simulink model "PIcontrol_smo"  (R2022a)
settings: Solver=VariableStepAuto  StartTime=0.0  StopTime=2.5  MaxStep=1e-4  MinStep=1e-6  RelTol=1e-6
undefined symbols (not defined in the file or in its folder): DiscIntNeverNeededParam
libraries: spsIGBTDiodeLib x6, simulink x3, mcbcontrolslib x1, spsDCVoltageSourceLib x1, spsPermanentMagnetSynchronousMachineLib x1, spspowerguiLib x1
settings Model: Creator=18527  LastModifiedBy=18527
settings SolverCC: ZeroCrossAlgorithm=Adaptive
settings DebuggingCC: IgnoredZcDiagnostic=none

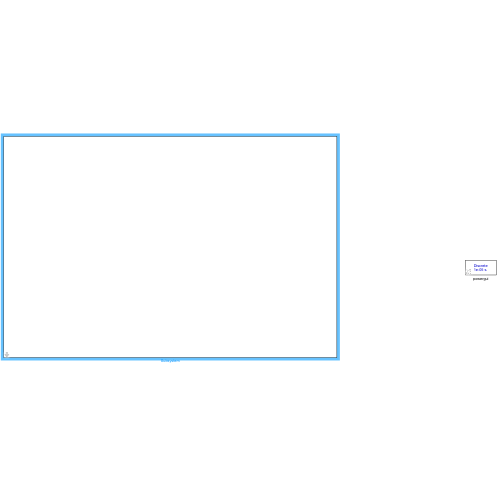
[thumbnail: Simulink's stored preview of the top-level diagram]
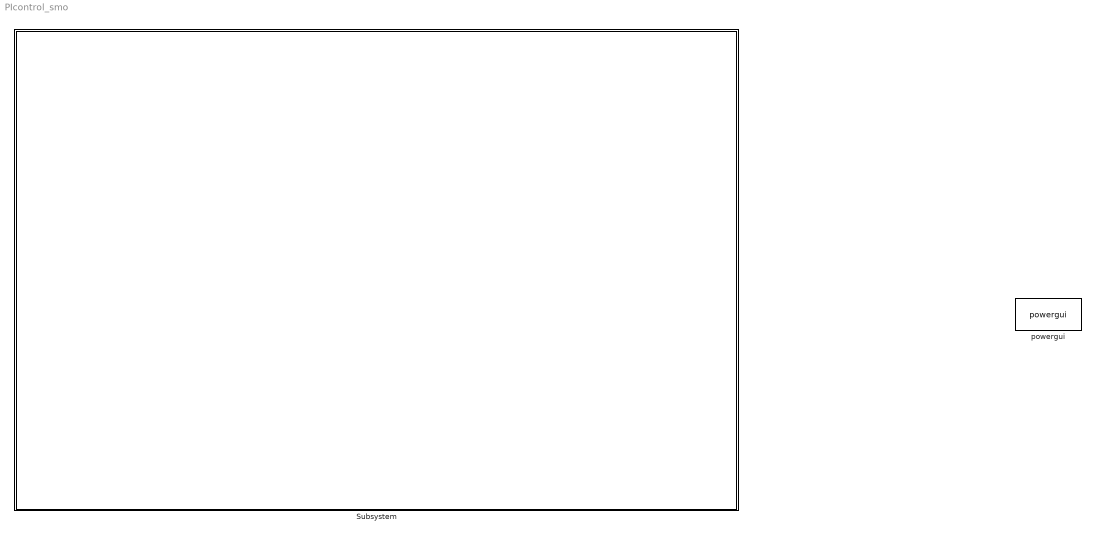
== system PIcontrol_smo ==
  Subsystem : Subsystem  mask{Pn=4, Ld=5.25e-3, Lq=12e-3, R=0.958, J=0.003, B=0.008, Phi=0.1827, OPL_Time=2, Switch_Speed=800}
      mask prompts: Pn "极对数"; Ld "定子电感"; Lq "定子电感"; R "定子电阻"; J "转动惯量"; B "阻尼系数"; Phi "磁链"; OPL_Time "开环时间"; Switch_Speed "切闭环速度"
      mask DialogControl ParameterGroupVar Prompt: 参数
  powergui : spspowerguiLib/powergui  Priority=1  SimulationMode=Discrete  SampleTime=1e-5  frequency=60  Iterations=50  frequencyindice=0  Pbase=100e6  ErrMax=1e-4  UnitsV=kV  UnitsW=MW  buscounter=0  FunctionMessages=off  echomessages=off  EnableUseOfTLC=off  CurrentSourceSwitches=off  DisableSnubberDevices=off  DisableRonSwitches=off  DisableVfSwitches=off  DisplayEquations=off  AutomaticDiscreteSolvers=off  SolverType=Tustin/Backward Euler (TBE)  Interpol=off  ExternalGateDelay=off  methode=off  Ts=100  x0status=blocks  SPID=on  SwTol=0  HookPort=off  NonlinearTolerance=1e-4  nMaxIteration=100  ContinueOnMaxIteration=off  RestoreLinks=warning  ResistiveCurrentMeasurement=off  Frange=[0:2:500]  Ylog=off  Xlog=on  ShowGrid=off  save=off  variable=ZData  structure=0  ZoomFFT=off  StartTime=0.0  cycles=1  DisplayStyle=1  fundamental=60  FreqAxis=off  MaxFrequency=1000  frequencyindicesteady=1  RmsSteady=1  display=off

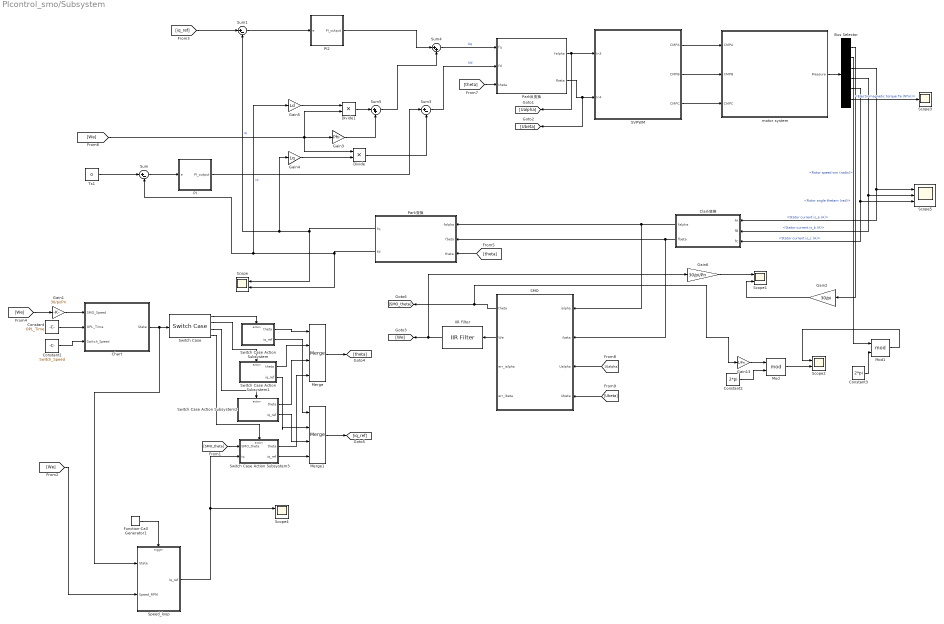
== system PIcontrol_smo/Subsystem ==
  Bus Selector : BusSelector  OutputSignals=Rotor speed wm (rad/s),Rotor angle thetam (rad),Stator current is_a (A),Stator current is_b (A),Stator current is_c (A),Electromagnetic torque Te (N*m)
  Chart : Stateflow chart  TreatAsAtomicUnit=on
  Clark变换 : Subsystem
  Constant : Constant  Value=OPL_Time
  Constant1 : Constant  Value=Switch_Speed
  Constant2 : Constant  Value=2*pi
  Constant3 : Constant  Value=2*pi
  Divide : Product  Inputs=**
  Divide1 : Product  Inputs=**
  Function-Call Generator1 : simulink/Ports & Subsystems/Function-Call Generator  sample_time=0.002  numberOfIterations=1  DisallowWideOutput=off
  Gain1 : Gain  Gain=30/pi/Pn
  Gain13 : Gain  Gain=1/Pn
  Gain2 : Gain  Gain=30/pi
  Gain3 : Gain  Gain=Phi
  Gain4 : Gain  Gain=Lq
  Gain5 : Gain  Gain=Ld
  Gain6 : Gain  Gain=30/pi/Pn
  IIR Filter : mcbcontrolslib/IIR Filter  VariantControl=Low Pass Filter  VariantSelect=Low-pass  Filter_constant=0.0008  advancedSettings=off  Ts=6e-6  cutOff_freq=21.2376
      settings: SourceProductBaseCode=MT
  Merge : Merge  Inputs=4
  Merge1 : Merge  Inputs=4
  Mod : Math  Operator=mod
  Mod1 : Math  Operator=mod
  PI : Subsystem  mask{Kp=Ld*4000/2, Ki=R*4000/2}
      mask prompts: Kp "比例"; Ki "积分"
      mask DialogControl ParameterGroupVar Prompt: 参数
  PI2 : Subsystem  mask{Kp=Lq*4000/2, Ki=R*4000/2}
      mask prompts: Kp "比例"; Ki "积分"
      mask DialogControl ParameterGroupVar Prompt: 参数
  Park反变换 : Subsystem
  Park变换 : Subsystem
  SMO : Subsystem
  SVPWM : Subsystem
  Scope{,1..2,4} (4 alike) : Scope  NumInputPorts=2
  Scope3 : Scope
  Scope5 : Scope  NumInputPorts=3
  Speed_loop : Subsystem
      settings: RTWSystemCode=Nonreusable function  RTWFcnNameOpts=Use subsystem name
  Sum : Sum  Inputs=|+-
  Sum1 : Sum  Inputs=|+-
  Sum3 : Sum  Inputs=|+-
  Sum4 : Sum  Inputs=|++
  Sum5 : Sum  Inputs=|++
  Switch Case : SwitchCase  CaseConditions={1,2,3,4}  ShowDefaultCase=off
  Switch Case Action Subsystem : Subsystem  TreatAsAtomicUnit=on
  Switch Case Action Subsystem1 : Subsystem  TreatAsAtomicUnit=on
  Switch Case Action Subsystem2 : Subsystem  TreatAsAtomicUnit=on
  Switch Case Action Subsystem3 : Subsystem  TreatAsAtomicUnit=on
  Ts1 : Constant  Value=0
  motor system : Subsystem
  wires:
  Sum1/1 -> PI2/1(e)
  Sum4/1 -> Park反变换/1(fq)  "Uq"
  motor system/1(Measure) -> Bus Selector/1
  PI2/1(PI_output) -> Sum4/1
  Park反变换/1(falpha) -> SVPWM/1(In3), [Ualpha]
  Park反变换/2(fbeta) -> [Ubeta], SVPWM/2(In4)
  SVPWM/1(CMPA) -> motor system/1(CMPA)
  SVPWM/2(CMPB) -> motor system/2(CMPB)
  SVPWM/3(CMPC) -> motor system/3(CMPC)
  Bus Selector/3 -> Scope5/1, Clark变换/1(fA)  "<Stator current is_a (A)>"
  Bus Selector/4 -> Clark变换/2(fB), Scope5/2  "<Stator current is_b (A)>"
  Bus Selector/5 -> Scope5/3, Clark变换/3(fC)  "<Stator current is_c (A)>"
  Clark变换/1(falpha) -> SMO/1(ialpha), Park变换/1(falpha)
  Clark变换/2(fbeta) -> SMO/2(ibeta), Park变换/2(fbeta)
  [Ubeta] -> SMO/4(Ubeta)
  [Ualpha] -> SMO/3(Ualpha)
  Gain5/1 -> Divide1/1
  [We] -> Divide1/2, Gain3/1, Divide/1
  PI/1(PI_output) -> Sum3/1
  Ts1/1 -> Sum/1
  Sum/1 -> PI/1(e)
  SMO/2(We) -> IIR Filter/1
  Gain4/1 -> Divide/2
  Park变换/2(fd) -> Scope/2, Gain5/1, Sum/2  "id"
  Park变换/1(fq) -> Scope/1, Gain4/1, Sum1/2  "iq"
  Divide1/1 -> Sum5/1
  Gain3/1 -> Sum5/2
  Divide/1 -> Sum3/2
  Sum5/1 -> Sum4/2
  Sum3/1 -> Park反变换/2(fd)  "Ud"
  Bus Selector/1 -> Gain2/1  "<Rotor speed wm (rad/s)>"
  Gain2/1 -> Scope1/2
  Gain6/1 -> Scope1/1
  SMO/1(theta) -> Gain13/1, [SMO_theta]
  Bus Selector/2 -> Mod1/1  "<Rotor angle thetam (rad)>"
  Bus Selector/6 -> Scope3/1  "<Electromagnetic torque Te (N*m)>"
  Switch Case/1 -> Switch Case Action Subsystem/Action
  Switch Case Action Subsystem/1(theta) -> Merge/1
  Switch Case/2 -> Switch Case Action Subsystem1/Action
  Switch Case/3 -> Switch Case Action Subsystem2/Action
  Switch Case Action Subsystem1/1(theta) -> Merge/2
  Switch Case Action Subsystem2/1(theta) -> Merge/3
  Switch Case Action Subsystem3/1(theta) -> Merge/4
  Switch Case Action Subsystem/2(iq_ref) -> Merge1/1
  Switch Case Action Subsystem1/2(iq_ref) -> Merge1/2
  Switch Case Action Subsystem2/2(iq_ref) -> Merge1/3
  Switch Case Action Subsystem3/2(iq_ref) -> Merge1/4
  Merge/1 -> [theta]
  Merge1/1 -> [iq_ref]
  IIR Filter/1 -> Gain6/1, [We]
  [SMO_theta] -> Switch Case Action Subsystem3/1(SMO_theta)
  [iq_ref] -> Sum1/1
  Switch Case/4 -> Switch Case Action Subsystem3/Action
  [We] -> Speed_loop/2(Speed_RPM)
  Chart/1(State) -> Speed_loop/1(State), Switch Case/1
  [We] -> Gain1/1
  Gain1/1 -> Chart/1(SMO_Speed)
  Constant/1 -> Chart/2(OPL_Time)
  Constant1/1 -> Chart/3(Switch_Speed)
  [theta] -> Park变换/3(theta)
  [theta] -> Park反变换/3(theta)
  Function-Call Generator1/1 -> Speed_loop/Trigger
  Speed_loop/1(Iq_ref) -> Scope4/1, Switch Case Action Subsystem3/2(iq)
  Constant2/1 -> Mod/2
  Mod/1 -> Scope2/2
  Gain13/1 -> Mod/1
  Constant3/1 -> Mod1/2
  Mod1/1 -> Scope2/1

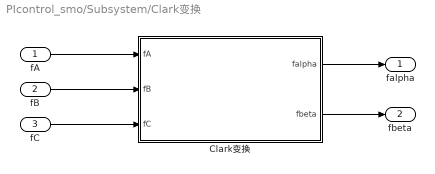
== system PIcontrol_smo/Subsystem/Clark变换 ==
  fA : Inport
  fB : Inport  Port=2
  fC : Inport  Port=3
  Clark变换 : MATLAB Function  TreatAsAtomicUnit=on
  falpha : Outport
  fbeta : Outport  Port=2
  wires:
  fB/1 -> Clark变换/2(fB)
  Clark变换/1(falpha) -> falpha/1
  fA/1 -> Clark变换/1(fA)
  fC/1 -> Clark变换/3(fC)
  Clark变换/2(fbeta) -> fbeta/1

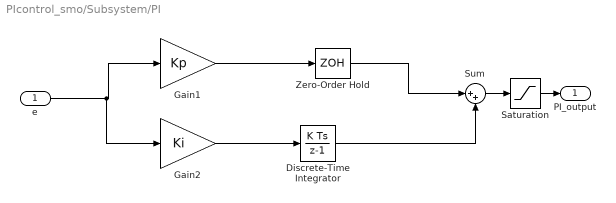
== system PIcontrol_smo/Subsystem/PI ==
  e : Inport
  Discrete-Time Integrator : DiscreteIntegrator  SampleTime=-1  ICPrevOutput=DiscIntNeverNeededParam  ICPrevScaledInput=DiscIntNeverNeededParam
  Gain1 : Gain  Gain=Kp
  Gain2 : Gain  Gain=Ki
  Saturation : Saturate  UpperLimit=sqrt(3)*311/3  LowerLimit=-sqrt(3)*311/3
  Sum : Sum  Inputs=|++
  Zero-Order Hold : ZeroOrderHold  SampleTime=-1
  PI_output : Outport
  wires:
  e/1 -> Gain2/1, Gain1/1
  Discrete-Time Integrator/1 -> Sum/2
  Gain2/1 -> Discrete-Time Integrator/1
  Zero-Order Hold/1 -> Sum/1
  Gain1/1 -> Zero-Order Hold/1
  Sum/1 -> Saturation/1
  Saturation/1 -> PI_output/1

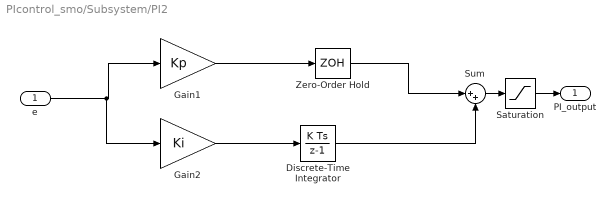
== system PIcontrol_smo/Subsystem/PI2 ==
  e : Inport
  Discrete-Time Integrator : DiscreteIntegrator  SampleTime=-1  ICPrevOutput=DiscIntNeverNeededParam  ICPrevScaledInput=DiscIntNeverNeededParam
  Gain1 : Gain  Gain=Kp
  Gain2 : Gain  Gain=Ki
  Saturation : Saturate  UpperLimit=sqrt(3)*311/3  LowerLimit=-sqrt(3)*311/3
  Sum : Sum  Inputs=|++
  Zero-Order Hold : ZeroOrderHold  SampleTime=-1
  PI_output : Outport
  wires:
  Gain1/1 -> Zero-Order Hold/1
  Zero-Order Hold/1 -> Sum/1
  Gain2/1 -> Discrete-Time Integrator/1
  Discrete-Time Integrator/1 -> Sum/2
  e/1 -> Gain1/1, Gain2/1
  Sum/1 -> Saturation/1
  Saturation/1 -> PI_output/1

== system PIcontrol_smo/Subsystem/Park反变换 ==
  fq : Inport
  fd : Inport  Port=2
  theta : Inport  Port=3
  Park反变换 : MATLAB Function  TreatAsAtomicUnit=on
  falpha : Outport
  fbeta : Outport  Port=2
  wires:
  fq/1 -> Park反变换/2(fq)
  Park反变换/1(falpha) -> falpha/1
  fd/1 -> Park反变换/1(fd)
  Park反变换/2(fbeta) -> fbeta/1
  theta/1 -> Park反变换/3(theta)

== system PIcontrol_smo/Subsystem/Park变换 ==
  falpha : Inport
  fbeta : Inport  Port=2
  theta : Inport  Port=3
  Park变换 : MATLAB Function  TreatAsAtomicUnit=on
  fq : Outport
  fd : Outport  Port=2
  wires:
  fbeta/1 -> Park变换/2(fbeta)
  Park变换/1(fd) -> fd/1
  falpha/1 -> Park变换/1(falpha)
  Park变换/2(fq) -> fq/1
  theta/1 -> Park变换/3(theta)

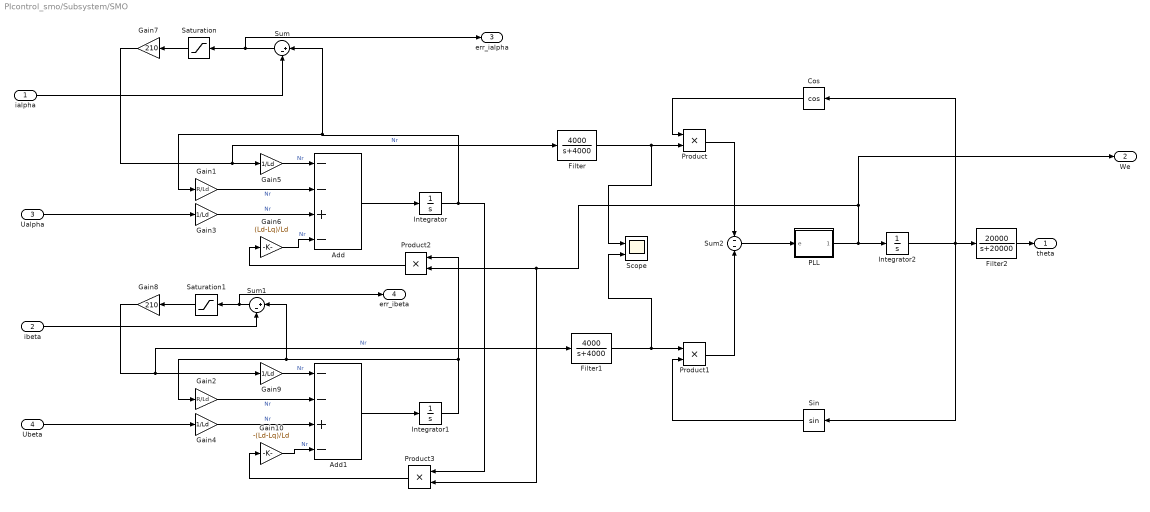
== system PIcontrol_smo/Subsystem/SMO ==
  ialpha : Inport
  ibeta : Inport  Port=2
  Ualpha : Inport  Port=3
  Ubeta : Inport  Port=4
  Add : Sum  Inputs=--+-
  Add1 : Sum  Inputs=--+-
  Cos : Trigonometry  Operator=cos
  Filter : TransferFcn  Numerator=[4000]  Denominator=[1 4000]
  Filter1 : TransferFcn  Numerator=[4000]  Denominator=[1 4000]
  Filter2 : TransferFcn  Numerator=[20000]  Denominator=[1 20000]
  Gain1 : Gain  Gain=R/Ld
  Gain10 : Gain  Gain=-(Ld-Lq)/Ld
  Gain2 : Gain  Gain=R/Ld
  Gain{3..5,9} (4 alike) : Gain  Gain=1/Ld
  Gain6 : Gain  Gain=(Ld-Lq)/Ld
  Gain7 : Gain  Gain=210
  Gain8 : Gain  Gain=210
  Integrator : Integrator
  Integrator1 : Integrator
  Integrator2 : Integrator
  PLL : Subsystem
      mask Display: disp('PI')
  Product{,1..3} (4 alike) : Product
  Saturation : Saturate  UpperLimit=1  LowerLimit=-1
  Saturation1 : Saturate  UpperLimit=1  LowerLimit=-1
  Scope : Scope  NumInputPorts=2
  Sin : Trigonometry
  Sum : Sum  Inputs=|+-
  Sum1 : Sum  Inputs=|+-
  Sum2 : Sum  Inputs=--
  theta : Outport
  We : Outport  Port=2
  err_ialpha : Outport  Port=3
  err_ibeta : Outport  Port=4
  wires:
  Gain1/1 -> Add/2  "Nr"
  Gain2/1 -> Add1/2  "Nr"
  Add/1 -> Integrator/1
  Integrator/1 -> Product3/1, Sum/1, Gain1/1
  Add1/1 -> Integrator1/1
  Integrator1/1 -> Product2/1, Sum1/1, Gain2/1
  Gain3/1 -> Add/3  "Nr"
  Ualpha/1 -> Gain3/1
  Ubeta/1 -> Gain4/1
  Gain4/1 -> Add1/3  "Nr"
  ialpha/1 -> Sum/2
  Gain5/1 -> Add/1  "Nr"
  ibeta/1 -> Sum1/2
  Saturation/1 -> Gain7/1
  Gain7/1 -> Filter/1, Gain5/1  "Nr"
  Sum1/1 -> err_ibeta/1, Saturation1/1
  Saturation1/1 -> Gain8/1
  Gain8/1 -> Filter1/1, Gain9/1  "Nr"
  Gain9/1 -> Add1/1  "Nr"
  Cos/1 -> Product/1
  Sin/1 -> Product1/2
  Product1/1 -> Sum2/2
  Product/1 -> Sum2/1
  Sum2/1 -> PLL/1(e)
  Integrator2/1 -> Sin/1, Filter2/1, Cos/1
  Product2/1 -> Gain6/1
  Gain6/1 -> Add/4  "Nr"
  Gain10/1 -> Add1/4  "Nr"
  Product3/1 -> Gain10/1
  Filter/1 -> Scope/1, Product/2
  Filter1/1 -> Scope/2, Product1/1
  Sum/1 -> err_ialpha/1, Saturation/1
  PLL/1(output) -> We/1, Product3/2, Product2/2, Integrator2/1
  Filter2/1 -> theta/1

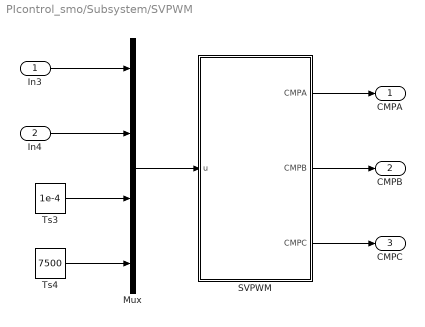
== system PIcontrol_smo/Subsystem/SVPWM ==
  In3 : Inport
  In4 : Inport  Port=2
  Mux : Mux
  SVPWM : MATLAB Function  TreatAsAtomicUnit=on
  Ts3 : Constant  Value=1e-4
  Ts4 : Constant  Value=7500
  CMPA : Outport
  CMPB : Outport  Port=2
  CMPC : Outport  Port=3
  wires:
  Mux/1 -> SVPWM/1(u)
  Ts4/1 -> Mux/4
  In4/1 -> Mux/2
  Ts3/1 -> Mux/3
  In3/1 -> Mux/1
  SVPWM/1(CMPA) -> CMPA/1
  SVPWM/2(CMPB) -> CMPB/1
  SVPWM/3(CMPC) -> CMPC/1

== system PIcontrol_smo/Subsystem/Speed_loop ==
  State : Inport
  Speed_RPM : Inport  Port=2
  function : TriggerPort  TriggerType=function-call  VariantControl=Variant
  Compare To Constant : simulink/Logic and Bit Operations/Compare To Constant  relop===  const=4  OutDataTypeStr=boolean
  SPD_Loop : Subsystem
  Iq_ref : Outport
  wires:
  State/1 -> Compare To Constant/1
  Speed_RPM/1 -> SPD_Loop/1(We)
  Compare To Constant/1 -> SPD_Loop/Enable
  SPD_Loop/1(iq) -> Iq_ref/1

== system PIcontrol_smo/Subsystem/Switch Case Action Subsystem ==
  Action Port : ActionPort  ActionPortLabel=case [ 1 ]:
  Constant : Constant  Value=0
  iq : Constant  Value=0
  theta : Outport
  iq_ref : Outport  Port=2
  wires:
  Constant/1 -> theta/1
  iq/1 -> iq_ref/1

== system PIcontrol_smo/Subsystem/Switch Case Action Subsystem1 ==
  Action Port : ActionPort  ActionPortLabel=case [ 2 ]:
  Constant : Constant  Value=-pi/2
  iq : Constant  Value=2
  theta : Outport
  iq_ref : Outport  Port=2
  wires:
  iq/1 -> iq_ref/1
  Constant/1 -> theta/1

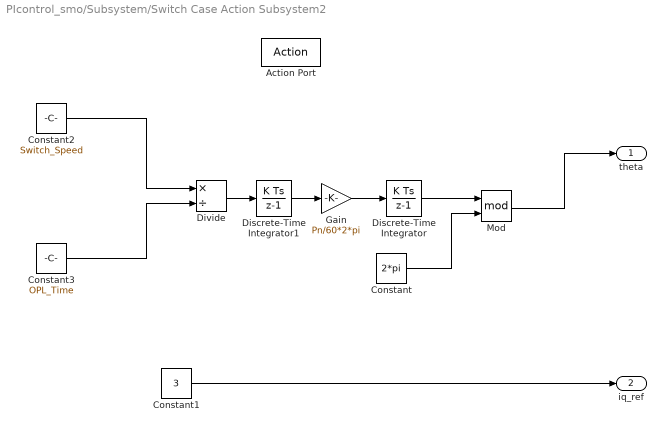
== system PIcontrol_smo/Subsystem/Switch Case Action Subsystem2 ==
  Action Port : ActionPort  ActionPortLabel=case [ 3 ]:
  Constant : Constant  Value=2*pi
  Constant1 : Constant  Value=3
  Constant2 : Constant  Value=Switch_Speed
  Constant3 : Constant  Value=OPL_Time
  Discrete-Time Integrator : DiscreteIntegrator  SampleTime=-1  ICPrevOutput=DiscIntNeverNeededParam  ICPrevScaledInput=DiscIntNeverNeededParam
  Discrete-Time Integrator1 : DiscreteIntegrator  SampleTime=-1  ICPrevOutput=DiscIntNeverNeededParam  ICPrevScaledInput=DiscIntNeverNeededParam
  Divide : Product  Inputs=*/
  Gain : Gain  Gain=Pn/60*2*pi
  Mod : Math  Operator=mod
  theta : Outport
  iq_ref : Outport  Port=2
  wires:
  Constant2/1 -> Divide/1
  Constant3/1 -> Divide/2
  Divide/1 -> Discrete-Time Integrator1/1
  Gain/1 -> Discrete-Time Integrator/1
  Discrete-Time Integrator1/1 -> Gain/1
  Discrete-Time Integrator/1 -> Mod/1
  Constant/1 -> Mod/2
  Mod/1 -> theta/1
  Constant1/1 -> iq_ref/1

== system PIcontrol_smo/Subsystem/Switch Case Action Subsystem3 ==
  SMO_theta : Inport
  iq : Inport  Port=2
  Action Port : ActionPort  ActionPortLabel=case [ 4 ]:
  theta : Outport
  iq_ref : Outport  Port=2
  wires:
  SMO_theta/1 -> theta/1
  iq/1 -> iq_ref/1

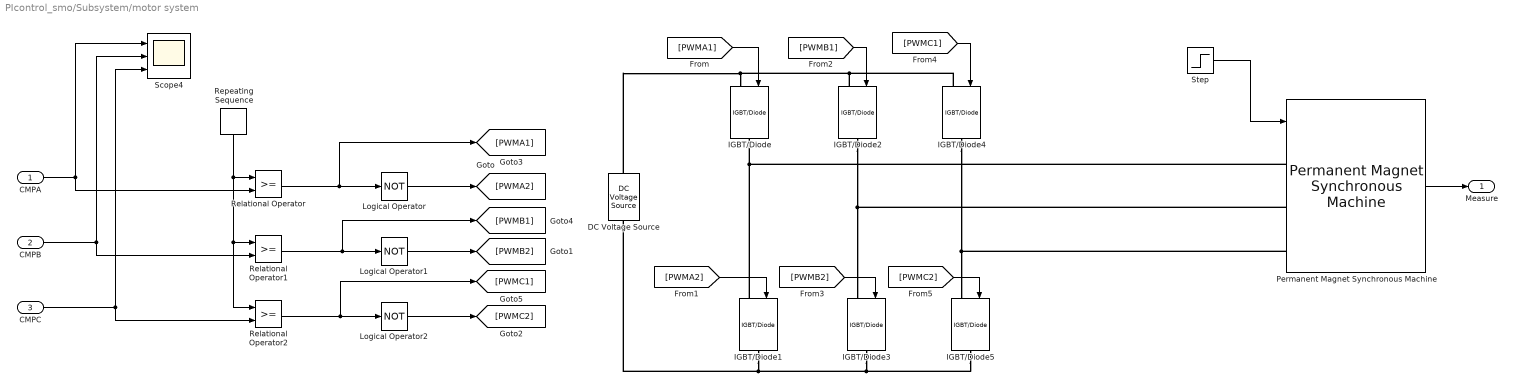
== system PIcontrol_smo/Subsystem/motor system ==
  CMPA : Inport
  CMPB : Inport  Port=2
  CMPC : Inport  Port=3
  DC Voltage Source : spsDCVoltageSourceLib/DC Voltage Source  Amplitude=311  Measurements=None
  IGBT/Diode{,1..5} (6 alike) : spsIGBTDiodeLib/IGBT//Diode  Ron=1e-3  Rs=1e5  Cs=inf  Measurements=off
  Logical Operator : Logic  Operator=NOT  AllPortsSameDT=off  OutDataTypeStr=boolean
  Logical Operator1 : Logic  Operator=NOT  AllPortsSameDT=off  OutDataTypeStr=boolean
  Logical Operator2 : Logic  Operator=NOT  AllPortsSameDT=off  OutDataTypeStr=boolean
  Permanent Magnet Synchronous Machine : spsPermanentMagnetSynchronousMachineLib/Permanent Magnet Synchronous Machine  NbPhases=3  FluxDistribution=Sinusoidal  RotorType=Salient-pole  MechanicalLoad=Torque Tm  PresetModel=No  ShowDetailedParameters=on  MeasurementBus=off  Resistance=R  Inductance=8.5e-3  dqInductances=[Ld,Lq]  La=0.000395  MachineConstant=Flux linkage established by magnets (V.s)  Flux=Phi  VoltageCst=132.5525  TorqueCst=1.0962  Flat=120  Mechanical=[J B 4]  PolePairs=4  InitialConditions=[0,0, 0,0]  InitialConditions5ph=[0 0 0 0 0 0]  RefAngle=Aligned with phase A axis (original Park)  IterativeDiscreteModel=Trapezoidal non iterative  TsBlock=-1  TsPowergui=0
  Relational Operator : RelationalOperator  OutDataTypeStr=boolean  RndMeth=Simplest  InputSameDT=off
  Relational Operator1 : RelationalOperator  OutDataTypeStr=boolean  RndMeth=Simplest  InputSameDT=off
  Relational Operator2 : RelationalOperator  OutDataTypeStr=boolean  RndMeth=Simplest  InputSameDT=off
  Repeating Sequence : simulink/Sources/Repeating Sequence  rep_seq_t=[0 5e-5 1e-4]  rep_seq_y=[0 7500 0]
  Scope4 : Scope  NumInputPorts=3
  Step : Step  Time=0.2  After=0  SampleTime=0
  Measure : Outport
  wires:
  [PWMC1] -> IGBT/Diode4/1
  [PWMA2] -> IGBT/Diode1/1
  [PWMB2] -> IGBT/Diode3/1
  [PWMC2] -> IGBT/Diode5/1
  [PWMA1] -> IGBT/Diode/1
  [PWMB1] -> IGBT/Diode2/1
  Logical Operator1/1 -> [PWMB2]
  Repeating Sequence/1 -> Relational Operator2/1, Relational Operator1/1, Relational Operator/1
  Relational Operator/1 -> [PWMA1], Logical Operator/1
  Relational Operator1/1 -> [PWMB1], Logical Operator1/1
  CMPC/1 -> Relational Operator2/2, Scope4/3
  Logical Operator/1 -> [PWMA2]
  CMPB/1 -> Relational Operator1/2, Scope4/2
  Logical Operator2/1 -> [PWMC2]
  CMPA/1 -> Relational Operator/2, Scope4/1
  Relational Operator2/1 -> [PWMC1], Logical Operator2/1
  Step/1 -> Permanent Magnet Synchronous Machine/1
  Permanent Magnet Synchronous Machine/1 -> Measure/1
  connections:
  IGBT/Diode1/LConn1 -- Permanent Magnet Synchronous Machine/LConn1 -- IGBT/Diode/RConn1
  IGBT/Diode1/RConn1 -- IGBT/Diode5/RConn1 -- IGBT/Diode3/RConn1 -- DC Voltage Source/LConn1
  IGBT/Diode/LConn1 -- IGBT/Diode4/LConn1 -- IGBT/Diode2/LConn1 -- DC Voltage Source/RConn1
  IGBT/Diode4/RConn1 -- Permanent Magnet Synchronous Machine/LConn3 -- IGBT/Diode5/LConn1
  IGBT/Diode2/RConn1 -- IGBT/Diode3/LConn1 -- Permanent Magnet Synchronous Machine/LConn2

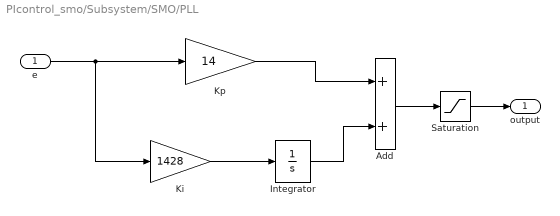
== system PIcontrol_smo/Subsystem/SMO/PLL ==
  e : Inport
  Add : Sum
  Integrator : Integrator
  Ki : Gain  Gain=1428
  Kp : Gain  Gain=14
  Saturation : Saturate  UpperLimit=1000  LowerLimit=-1000
  output : Outport
  wires:
  Add/1 -> Saturation/1
  Kp/1 -> Add/1
  Integrator/1 -> Add/2
  Saturation/1 -> output/1
  e/1 -> Ki/1, Kp/1
  Ki/1 -> Integrator/1

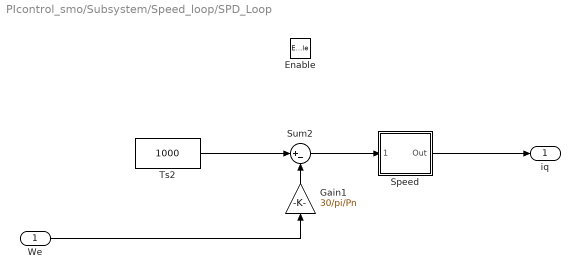
== system PIcontrol_smo/Subsystem/Speed_loop/SPD_Loop ==
  We : Inport
  Enable : EnablePort
  Gain1 : Gain  Gain=30/pi/Pn
  Speed : Subsystem  AncestorBlock=|  DialogController=POWERSYS.PowerSysDialog  mask(Discrete PI Controller){Kp=0.038, Ki=1, Par_Limits=[25 -25], Init=0}
      | powerlib_extras/Discrete 
      | Control Blocks/Discrete
      | PI Controller
      mask prompts: Kp "Proportional gain (Kp):"; Ki "Integral gain (Ki):"; Par_Limits "Output limits: [ Upper   Lower ]"; Init "Output initial value:"
      mask help: This block implements a discrete PI controller.
      mask init:
      | UpperLimit=Par_Limits(1);
      | LowerLimit=Par_Limits(2);
      | power_initmask();
      mask Help: This block is part of a subset of blocks in the Extras library that does not have documentation associated with it, other than the block mask description.
      mask Display: disp('PI');
  Sum2 : Sum  Inputs=|+-
  Ts2 : Constant  Value=1000
  iq : Outport
  wires:
  We/1 -> Gain1/1
  Speed/1(Out) -> iq/1
  Ts2/1 -> Sum2/1
  Gain1/1 -> Sum2/2
  Sum2/1 -> Speed/1(Error)

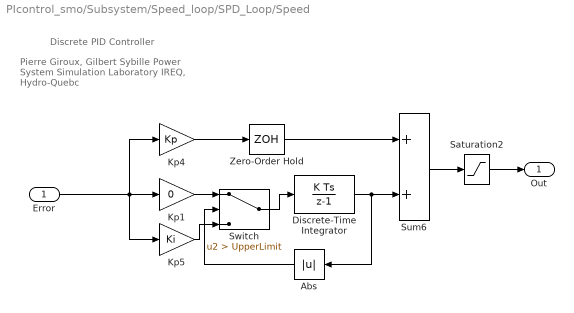
== system PIcontrol_smo/Subsystem/Speed_loop/SPD_Loop/Speed ==
  note: Discrete PID Controller
  note: Pierre Giroux, Gilbert Sybille
      | Power System Simulation Laboratory
      | IREQ, Hydro-Quebc
  Error : Inport
  Abs : Abs  SaturateOnIntegerOverflow=off
  Discrete-Time Integrator : DiscreteIntegrator  InitialCondition=Init  SampleTime=-1  LimitOutput=on  UpperSaturationLimit=UpperLimit  LowerSaturationLimit=LowerLimit  ICPrevOutput=DiscIntNeverNeededParam  ICPrevScaledInput=DiscIntNeverNeededParam
  Kp1 : Gain  Gain=0  SaturateOnIntegerOverflow=on  OutDataTypeStr=Inherit: Same as input  ParamDataTypeStr=Inherit: Same as input
  Kp4 : Gain  Gain=Kp  SaturateOnIntegerOverflow=on  OutDataTypeStr=Inherit: Same as input  ParamDataTypeStr=Inherit: Same as input
  Kp5 : Gain  Gain=Ki  SaturateOnIntegerOverflow=on  OutDataTypeStr=Inherit: Same as input  ParamDataTypeStr=Inherit: Same as input
  Saturation2 : Saturate  UpperLimit=UpperLimit  LowerLimit=LowerLimit
  Sum6 : Sum  InputSameDT=on  SaturateOnIntegerOverflow=on  OutDataTypeStr=Inherit: Same as first input
  Switch : Switch  Criteria=u2 > Threshold  Threshold=UpperLimit  SaturateOnIntegerOverflow=off  InputSameDT=off
  Zero-Order Hold : ZeroOrderHold  SampleTime=-1
  Out : Outport  InitialOutput=0  VectorParamsAs1DForOutWhenUnconnected=off
  wires:
  Zero-Order Hold/1 -> Sum6/1
  Saturation2/1 -> Out/1
  Discrete-Time Integrator/1 -> Abs/1, Sum6/2
  Kp4/1 -> Zero-Order Hold/1
  Sum6/1 -> Saturation2/1
  Error/1 -> Kp4/1, Kp1/1, Kp5/1
  Switch/1 -> Discrete-Time Integrator/1
  Abs/1 -> Switch/2
  Kp5/1 -> Switch/3
  Kp1/1 -> Switch/1

== matlab function PIcontrol_smo/Subsystem/Clark变换/Clark变换 ==
  data: fA input; falpha output; fB input; fC input; fbeta output
function [falpha,fbeta] = fcn(fA,fB,fC)
fABC = [fA fB fC]';
N = 2/3;%等幅值变换
T3sto2s = [1 -1/2 -1/2;0 sqrt(3)/2 -sqrt(3)/2;sqrt(2)/2 sqrt(2)/2 sqrt(2)/2];
temp = N*T3sto2s * fABC;
falpha = temp(1);
fbeta = temp(2);
end

== matlab function PIcontrol_smo/Subsystem/SVPWM/SVPWM ==
  data: u input; CMPA output; CMPB output; CMPC output
function [CMPA, CMPB, CMPC] = SVPWM(u)
Valpha = u(1);
Vbeta = u(2);
% Vc = u(3);
Ts = u(3);
PRD = u(4);


%60°坐标变换

Vg = Valpha - (1/sqrt(3))*Vbeta;
Vh = 2*Vbeta/sqrt(3);

%标幺化
Vdc = 311;
Vg = Vg/(2*Vdc/3);
Vh = Vh/(2*Vdc/3);

%判断扇区

if(Vh >= 0 && Vg >= 0)
    Sec = 1;
    Vgg = Vg;
    Vhh = Vh;
elseif(Vh >= 0 && Vg + Vh >= 0)
    Sec = 2;
    Vgg = -Vg;
    Vhh = Vg + Vh;
elseif(Vh >= 0 && Vg + Vh <= 0)
    Sec = 3;
    Vgg = Vh;
    Vhh = -Vg - Vh;
elseif(Vg <=0 && Vh <= 0)
    Sec = 4;
    Vgg = -Vh;
    Vhh = -Vg;
elseif(Vg >= 0 && Vg + Vh <= 0)
    Sec = 5;
    Vgg = -Vg - Vh;
    Vhh = Vg;
else
    Sec = 6;
    Vhh = -Vh;
    Vgg = Vg + Vh;
end
%计算T0，T1，T2矢量作用的时间

T1 = Vgg;
T2 = Vhh;
T0 = 1 - T1 - T2;

if(T0 < 0)
    Tsum = T1 + T2;
    T1 = T1 / Tsum;
    T2 = T2 / Tsum;
    T0 = 0;
end

TL = 0.25 * T0;
TM = TL + 0.5 * T1;
TH = TM + 0.5 * T2;

CL = TL * PRD * 2;
CM = TM * PRD * 2;
CH = TH * PRD * 2;
switch Sec
    case 1
        CMPA = CL;
        CMPB = CM;
        CMPC = CH;
    case 2
        CMPA = CM;
        CMPB = CL;
        CMPC = CH;
    case 3
        CMPA = CH;
        CMPB = CL;
        CMPC = CM;
    case 4
        CMPA = CH;
        CMPB = CM;
        CMPC = CL;
    case 5
        CMPA = CM;
        CMPB = CH;
        CMPC = CL;
    case 6
        CMPA = CL;
        CMPB = CH;
        CMPC = CM;
    otherwise 
        CMPA = CL;  % 不会进入这个分支，但是matlab要求必须有 otherwise
        CMPB = CH;
        CMPC = CM;    
end

== matlab function PIcontrol_smo/Subsystem/Park变换/Park变换 ==
  data: falpha input; fd output; fbeta input; fq output; theta input
function [fd,fq] = fcn(falpha, fbeta, theta)
f2s = [falpha fbeta]';
T2sto2r = [cos(theta) sin(theta);-sin(theta) cos(theta)];
temp = T2sto2r * f2s;
fd = temp(1);
fq = temp(2);
end

== matlab function PIcontrol_smo/Subsystem/Park反变换/Park反变换 ==
  data: fd input; falpha output; fq input; fbeta output; theta input
function [falpha,fbeta] = fcn(fd, fq, theta)
f2r = [fd fq]';
T2rto2s = [cos(theta) -sin(theta);sin(theta) cos(theta)];
temp = T2rto2s * f2r;
falpha = temp(1);
fbeta = temp(2);
end

== stateflow chart PIcontrol_smo/Subsystem/Chart ==
  state start
    State = 1;
  state align_angle
    State = 2
  state openloop
    State = 3;
  state closeloop
    State = 4;
  (default) -> start
  start -> align_angle
  align_angle -> openloop : [after(1,msec)]
  openloop -> closeloop : [after(OPL_Time,sec) && SMO_Speed > Switch_Speed ]
  data: SMO_Speed input; State output; OPL_Time input; Switch_Speed input
